simulink model "sm_boom_lift_crawler"  (R2026a)
settings: Solver=ode23t  StopTime=tVec.StopTime  FixedStep=2e-3  MaxStep=2  AbsTol=1e-3
StartFcn:
  | tic;
StopFcn:
  | Elapsed_Sim_Time = toc;
  | %disp(['Elapsed Sim Time = ' num2str(Elapsed_Sim_Time)]);
undefined symbols (not defined in the file): BasketR, Boom, Chassis, Extend, Jib, LevelM, LevelS, Lift, operator_seq, OutFL, OutFR, OutRL, OutRR, oVec, Tilt, TrackL, TrackR, Turret, tVec
libraries: sm_boom_lift_crawler_lib x14, nesl_utility x2, sm_lib x2, sm_boom_lift_crawler_lib_actuators x1, sm_boom_lift_crawler_lib_control x1, sm_boom_lift_crawler_lib_lift x1
(part 1 of 2)
Description:
  | Boom Lift Crawler with Hydraulic Actuation
  | 
  | Copyright 2020-2026 The MathWorks, Inc.
settings Model: Creator=smiller  LastModifiedBy=smiller
settings SolverCC: MaxConsecutiveMinStep=10
settings DataIOCC: SignalLoggingName=logsout_sm_boom_lift_crawler
settings SimscapeCC: SimscapeNominalValues="[{\"value\":\"1\",\"unit\":\"A\"},{\"value\":\"nomval_psi\",\"unit\":\"psi\"},{\"value\":\"1\",\"unit\":\"cm^2\"},{\"value\":\"nomval_cmv3_s\",\"unit\":\"cm^3/s\"},{\"value\":\"1\",\"unit\":\"kJ/kg\"},{\"value\":\"1\",\"unit\":\"kW\"},{\"value\":\"1\",\"unit\":\"l\"},{\"value\":\"nomval_N\",\"unit\":\"N\"},{\"value\":\"nomval_Nm\",\"unit\":\"N*m\"},{\"value\":\"1\",\"unit\":\"V\"}]"  SimscapeLogName=simlog_sm_boom_lift_crawler  SimscapeLogLimitData=off  SimscapeLogDataHistory=5000.0  SimscapeUseOperatingPoints=on  SimscapeOperatingPoint=op_hold15Sec_FULL
settings DiagnosticsConfigSet: SimMechanicsConflictingReferenceFrames=none  SimMechanicsRigidlyBoundBlock=none  SimMechanicsUnsatisfiedHighPriorityTargets=none
settings ExplorerConfigSet: InternalSimMechanicsExplorerSettings="<ExplorerConfiguration><canonicalview>default</canonicalview><AnimationSetting><BasePlaybackSpeed>1.0</BasePlaybackSpeed><PlaybackSpeedFactor>8.0</PlaybackSpeedFactor></AnimationSetting><TilePanel><TileInfo><Tiles Columns=\"1\" Count=\"1\" Rows=\"1\"><Column Weight=\"1\"/><Row Weight=\"1\"/><Tile Height=\"1\" Width=\"1\" X=\"0\" Y=\"0\"/></Tiles></TileInfo><SceneInfo><SceneViewer><BGColor><R>1</R><G>1</G><B>1</B></BGColor><Camera><DoPerspective>on</DoPerspective><Position><X>-12.2424581714389937</X><Y>-0.143345264209557399</Y><Z>4.1505972342390427</Z></Position><Center><X>-4.62122899968606404</X><Y>-0.143345264209557399</Y><Z>4.15059723423904359</Z></Center><Up><X>0</X><Y>0</Y><Z>1</Z></Up><ViewLimDist>1</ViewLimDist><YLim>0.466307658154998583</YLim><XLim>0.828991392275552963</XLim></Camera></SceneViewer></SceneInfo></TilePanel><MechEditorPanel><Cameras><Camera><Id>Camera8</Id><Value><Name>Extend_Knuckle</Name><NativeCamera><PositionTrackingFeature>Lift.Boom.Arms.Telescope.Extend_Cylinder.Transform_Camera_Extend_Knuckle.F</PositionTrackingFeature><CenterTrackingFeature>Lift.Boom.Arms.Telescope.Extend_Cylinder.Transform_Camera_Extend_Knuckle.F</CenterTrackingFeature><UpVectorTrackingFeature>Lift.Boom.Arms.Telescope.Extend_Cylinder.Transform_Camera_Extend_Knuckle.F</UpVectorTrackingFeature><CenterTrackingOrigin>off</CenterTrackingOrigin><CenterTrackingDirection>-X</CenterTrackingDirection><UpVectorTrackingDirection>-Y</UpVectorTrackingDirection></NativeCamera></Value></Camera><Camera><Id>Camera9</Id><Value><Name>Extend_Basket</Name><NativeCamera><PositionTrackingFeature>Lift.Boom.Arms.Telescope.Extend_Cylinder.Transform_Camera_Extend_Basket.F</PositionTrackingFeature><CenterTrackingFeature>Lift.Boom.Arms.Telescope.Extend_Cylinder.Transform_Camera_Extend_Basket.F</CenterTrackingFeature><UpVectorTrackingFeature>Lift.Boom.Arms.Telescope.Extend_Cylinder.Transform_Camera_Extend_Basket.F</UpVectorTrackingFeature><CenterTrackingOrigin>off</CenterTrackingOrigin><CenterTrackingDirection>+X</CenterTrackingDirection><UpVectorTrackingDirection>+Y</UpVectorTrackingDirection></NativeCamera></Value></Camera><Camera><Id>Camera10</Id><Value><Name>Basket_Rotate</Name><NativeCamera><PositionTrackingFeature>Lift.Boom.Basket.Basket_Rotate.Bracket.Reference_Camera_Basket_Rotate_L.R</PositionTrackingFeature><CenterTrackingFeature>Lift.Boom.Basket.Basket_Rotate.Bracket.Reference_Camera_Basket_Rotate_L.R</CenterTrackingFeature><UpVectorTrackingFeature>Mech_Config.World.W</UpVectorTrackingFeature><CenterTrackingOrigin>off</CenterTrackingOrigin><CenterTrackingDirection>-X</CenterTrackingDirection><UpVectorTrackingDirection>+Z</UpVectorTrackingDirection></NativeCamera></Value></Camera><Camera><Id>Camera11</Id><Value><Name>Tilt_Knuckle</Name><NativeCamera><PositionTrackingFeature>Lift.Boom.Arms.Tower.Upper_Knuckle.Reference_Knuckle_Cam.R</PositionTrackingFeature><CenterTrackingFeature>Lift.Boom.Arms.Tower.Upper_Knuckle.Reference_Knuckle_Cam.R</CenterTrackingFeature><UpVectorTrackingFeature>Mech_Config.World.W</UpVectorTrackingFeature><CenterTrackingOrigin>off</CenterTrackingOrigin><CenterTrackingDirection>+Z</CenterTrackingDirection><UpVectorTrackingDirection>+Z</UpVectorTrackingDirection></NativeCamera></Value></Camera><Camera><Id>Camera12</Id><Value><Name>Full Test</Name><NativeCamera><PositionKeyframeSet><Keyframe><Time>0</Time><Value><X>-12.242458171438994</X><Y>-0.1433452642095574</Y><Z>4.1505972342390427</Z></Value></Keyframe><Keyframe><Time>69.026826430124729</Time><Value><X>-14.974593328379619</X><Y>0.0056652615564253064</Y><Z>5.3389029552684786</Z></Value></Keyframe><Keyframe><Time>110.29539843687829</Time><Value><X>-21.00761369699504</X><Y>-0.0057417156870510078</Y><Z>8.0689402037867488</Z></Value></Keyframe><Keyframe><Time>140.70430157635164</Time><Value><X>-31.272784439198116</X><Y>-2.5583130214499052e-10</Y><Z>12.723321478963756</Z></Value></Keyframe><Keyframe><Time>181.77628976806102</Time><Value><X>-31.272784439198116</X><Y>-2.5583130214499052e-10</Y><Z>12.723321478963756</Z></Value></Keyframe><Keyframe><Time>208.0087867386398</Time><Value><X>-23.351505250921551</X><Y>-2.5583182919801497e-10</Y><Z>9.1371534281977738</Z></Value></Keyframe><Keyframe><Time>243.06358572448306</Time><Value><X>-16.577121762622586</X><Y>-2.5583144573665537e-10</Y><Z>6.0702143126734844</Z></Value></Keyframe><Keyframe><Time>273.3415757110605</Time><Value><X>-16.577121762622586</X><Y>-2.5583144573665537e-10</Y><Z>6.0702143126734844</Z></Value></Keyframe><Keyframe><Time>321.2447002217541</Time><Value><X>-13.690590902490033</X><Y>0.01787769923724114</Y><Z>4.7891626503614262</Z></Value></Keyframe><Keyframe><Time>350</Time><Value><X>-13.690590902490033</X><Y>0.01787769923724114</Y><Z>4.7891626503614262</Z></Value></Keyframe></PositionKeyframeSet><CenterKeyframeSet><Keyframe><Time>0</Time><Value><X>-4.621228999686064</X><Y>-0.1433452642095574</Y><Z>4.1505972342390436</Z></Value></Keyframe><Keyframe><Time>69.026826430124729</Time><Value><X>-0.17395018713353672</X><Y>0.0056652615564253064</Y><Z>5.3389029552684786</Z></Value></Keyframe><Keyframe><Time>110.29539843687829</Time><Value><X>-9.0038066291239502</X><Y>-0.0057417156870549491</Y><Z>8.0689402037867524</Z></Value></Keyframe><Keyframe><Time>140.70430157635164</Time><Value><X>-14.136391845814327</X><Y>-2.5583979379462107e-10</Y><Z>12.72332147896376</Z></Value></Keyframe><Keyframe><Time>181.77628976806102</Time><Value><X>-2.3429975002054775</X><Y>-2.5584563781180217e-10</Y><Z>12.723321478963761</Z></Value></Keyframe><Keyframe><Time>208.0087867386398</Time><Value><X>-10.17575261115104</X><Y>-2.5583801743778167e-10</Y><Z>9.1371534281977755</Z></Value></Keyframe><Keyframe><Time>243.06358572448306</Time><Value><X>-0.54476849060194255</X><Y>-2.5583897563257738e-10</Y><Z>6.0702143126734844</Z></Value></Keyframe><Keyframe><Time>273.3415757110605</Time><Value><X>-0.11057247639663359</X><Y>-2.5583917956089291e-10</Y><Z>6.0702143126734844</Z></Value></Keyframe><Keyframe><Time>321.2447002217541</Time><Value><X>-5.3452949964231387</X><Y>0.017877699237237366</Y><Z>4.7891626503614253</Z></Value></Keyframe><Keyframe><Time>350</Time><Value><X>-5.3452949964231387</X><Y>0.017877699237237366</Y><Z>4.7891626503614253</Z></Value></Keyframe></CenterKeyframeSet><UpVectorKeyframeSet><Keyframe><Time>0</Time><Value><X>0</X><Y>0</Y><Z>1</Z></Value></Keyframe><Keyframe><Time>69.026826430124729</Time><Value><X>0</X><Y>0</Y><Z>1</Z></Value></Keyframe><Keyframe><Time>110.29539843687829</Time><Value><X>0</X><Y>0</Y><Z>1</Z></Value></Keyframe><Keyframe><Time>140.70430157635164</Time><Value><X>0</X><Y>0</Y><Z>1</Z></Value></Keyframe><Keyframe><Time>181.77628976806102</Time><Value><X>-2.0731981129868445e-16</X><Y>1.0273382740432149e-31</Y><Z>1</Z></Value></Keyframe><Keyframe><Time>208.0087867386398</Time><Value><X>1.4663775813922931e-57</X><Y>2.9591920320379324e-42</Y><Z>1</Z></Value></Keyframe><Keyframe><Time>243.06358572448306</Time><Value><X>1.3898401336634517e-57</X><Y>2.9591920320379324e-42</Y><Z>1</Z></Value></Keyframe><Keyframe><Time>273.3415757110605</Time><Value><X>1.3898401336605064e-57</X><Y>2.9591920320379324e-42</Y><Z>1</Z></Value></Keyframe><Keyframe><Time>321.2447002217541</Time><Value><X>1.3198478700492623e-57</X><Y>2.9591920320379324e-42</Y><Z>1</Z></Value></Keyframe><Keyframe><Time>350</Time><Value><X>1.0642863113510858e-16</X><Y>-4.813997747953607e-32</Y><Z>1</Z></Value></Keyframe></UpVectorKeyframeSet></NativeCamera></Value></Camera><Camera><Id>Camera13</Id><Value><Name>View_Basket_World</Name><NativeCamera><PositionTrackingFeature>Lift.Boom.Basket.Basket.Reference_Basket_Cam.R</PositionTrackingFeature><CenterTrackingFeature>Mech_Config.World.W</CenterTrackingFeature><UpVectorTrackingFeature>Lift.Boom.Basket.Basket.Reference_Basket_Cam.R</UpVectorTrackingFeature><CenterTrackingOrigin>on</CenterTrackingOrigin><UpVectorTrackingDirection>+Y</UpVectorTrackingDirection></NativeCamera></Value></Camera><Camera><Id>Camera14</Id><Value><Name>View_Worm_Drive</Name><NativeCamera><PositionTrackingFeature>Lift.Boom.Turret.Case.Reference_Worm_Cam.R</PositionTrackingFeature><CenterTrackingFeature>Lift.Boom.Turret.Case.Transform_Worm_Cam.B</CenterTrackingFeature><UpVectorTrackingFeature>Mech_Config.World.W</UpVectorTrackingFeature><CenterTrackingOrigin>on</CenterTrackingOrigin><UpVectorTrackingDirection>+Z</UpVectorTrackingDirection></NativeCamera></Value></Camera><Camera><Id>Camera15</Id><Value><Name>Extend_Retract_Pulley</Name><NativeCamera><PositionTrackingFeature>Lift.Boom.Arms.Telescope.Extend_Cylinder.Reference_Camera_Retract_Pulley.R</PositionTrackingFeature><CenterTrackingFeature>Lift.Boom.Arms.Telescope.Extend_Cylinder.Reference_Camera_Retract_Pulley.R</CenterTrackingFeature><UpVectorTrackingFeature>Lift.Boom.Arms.Telescope.Extend_Cylinder.Reference_Camera_Retract_Pulley.R</UpVectorTrackingFeature><CenterTrackingOrigin>off</CenterTrackingOrigin><CenterTrackingDirection>+Y</CenterTrackingDirection><UpVectorTrackingDirection>+Z</UpVectorTrackingDirection></NativeCamera></Value></Camera><Camera><Id>Camera16</Id><Value><Name>Extend_Extend_Pulley</Name><NativeCamera><PositionTrackingFeature>Lift.Boom.Arms.Telescope.Extend_Cylinder.Reference_Camera_Extend_Pulley.R</PositionTrackingFeature><CenterTrackingFeature>Lift.Boom.Arms.Telescope.Extend_Cylinder.Reference_Camera_Extend_Pulley.R</CenterTrackingFeature><UpVectorTrackingFeature>Lift.Boom.Arms.Telescope.Extend_Cylinder.Reference_Camera_Extend_Pulley.R</UpVectorTrackingFeature><CenterTrackingOrigin>off</CenterTrackingOrigin><CenterTrackingDirection>+Z</CenterTrackingDirection><UpVectorTrackingDirection>-Y</UpVectorTrackingDirection></NativeCamera></Value></Camera><Camera><Id>Camera17</Id><Value><Name>Jib</Name><NativeCamera><PositionTrackingFeature>Lift.Boom.Basket.Jib.Jib_Mount.Reference_Camera_Basket_Jib.R</PositionTrackingFeature><CenterTrackingFeature>Lift.Boom.Basket.Jib.Jib_Mount.Reference_Camera_Basket_Jib.R</CenterTrackingFeature><UpVectorTrackingFeature>Mech_Config.World.W</UpVectorTrackingFeature><CenterTrackingOrigin>off</CenterTrackingOrigin><CenterTrackingDirection>-X</CenterTrackingDirection><UpVectorTrackingDirection>+Z</UpVectorTrackingDirection></NativeCamera></Value></Camera></Cameras><GfxPanelCameraMap><MapElement CameraMLId=\"Camera12\" GfxPanelIndex=\"0\"/></GfxPanelCameraMap><VideoCreator><PlaybackSpeedRatio>8</PlaybackSpeedRatio><FrameRate>30</FrameRate><VideoFormat>MPEG-4</VideoFormat><FrameSize>auto</FrameSize></VideoCreator></MechEditorPanel></ExplorerConfiguration>"

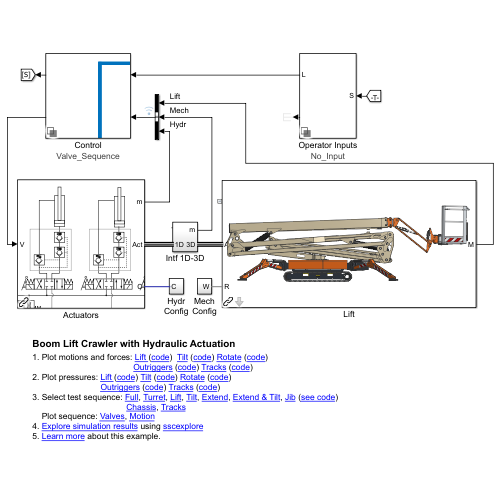
[thumbnail: Simulink's stored preview of the top-level diagram]
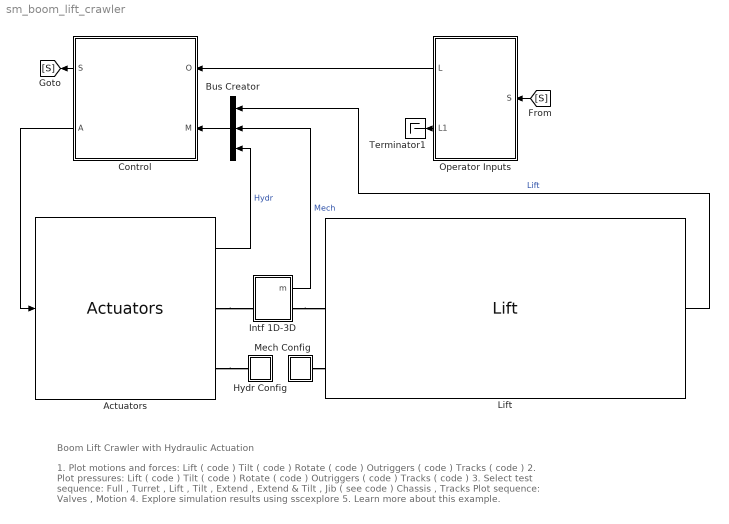
== system sm_boom_lift_crawler ==
  note: 1. Plot motions and forces: Lift ( code ) Tilt ( code ) Rotate ( code )
      | Outriggers ( code ) Tracks ( code )
      | 2. Plot pressures: Lift ( code ) Tilt ( code ) Rotate ( code )
      | Outriggers ( code ) Tracks ( code )
      | 3. Select test sequence: Full , Turret , Lift , Tilt , Extend , Extend & Tilt , Jib ( see code )
      | Chassis , Tracks
      | Plot sequence: Valves , Motion
      | 4. Explore simulation results using sscexplore
      | 5. Learn more about this example.
  note: Boom Lift Crawler with Hydraulic Actuation
  Actuators : sm_boom_lift_crawler_lib_actuators/Actuators  SystemSampleTime=-1  VariantControl=Actuators_CVs  VariantActivationTime=update diagram  EmptyChoice=off  PassThrough=off  PassThroughVariantControl=(default)  EmptyChoiceVariantControl=(default)  AllowFlexibleInterface=on  Latency=0  AutoFrameSizeCalculation=off
  Bus Creator : BusCreator  Inputs=3
  Control : Subsystem  Variant=on  VariantControlMode=label  VariantControl=Variant1  LabelModeActiveChoice=Valve_Sequence
      settings: AttributesFormatString=%<LabelModeActiveChoice>
      mask Display:
      | blk = sm_boom_lift_activeVariantBlock(gcb);
      | eval(get_param(blk, 'MaskDisplay'));
  Hydr Config : Subsystem
  Intf 1D-3D : Subsystem
  Lift : sm_boom_lift_crawler_lib_lift/Lift  popup_gnd_outr=Force
  Mech Config : Subsystem
  Operator Inputs : Subsystem  Variant=on  VariantControlMode=label  VariantControl=Variant1  LabelModeActiveChoice=No_Input
      settings: AttributesFormatString=%<LabelModeActiveChoice>
      mask Display:
      | blk = sm_boom_lift_activeVariantBlock(gcb);
      | eval(get_param(blk, 'MaskDisplay'));
  Terminator1 : Terminator
  wires:
  Control/2(A) -> Actuators/1
  Operator Inputs/1(L) -> Control/1(O)
  Actuators/1 -> Bus Creator/3  "Hydr"
  Intf 1D-3D/1(m) -> Bus Creator/2  "Mech"
  Bus Creator/1 -> Control/2(M)
  Lift/1 -> Bus Creator/1  "Lift"
  Operator Inputs/2(L1) -> Terminator1/1
  [S] -> Operator Inputs/1(S)
  Control/1(S) -> [S]
  connections:
  Mech Config/LConn1 -- Lift/LConn3
  Intf 1D-3D/RConn1 -- Lift/LConn2
  Actuators/RConn1 -- Intf 1D-3D/LConn2
  Actuators/RConn2 -- Hydr Config/RConn1

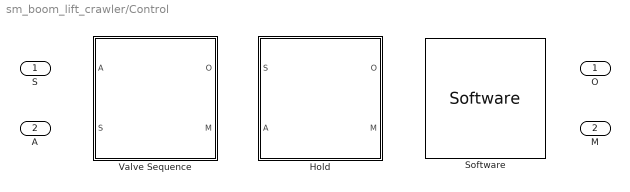
== system sm_boom_lift_crawler/Control ==
  O : Inport
  M : Inport  Port=2
  Hold : Subsystem  VariantControl=Hold
      mask Display: image('sm_boom_lift_crawler_valve_seq_hold.svg');
  Software : sm_boom_lift_crawler_lib_control/Software  SystemSampleTime=-1  VariantControl=Software  VariantActivationTime=update diagram  EmptyChoice=off  PassThrough=off  PassThroughVariantControl=(default)  EmptyChoiceVariantControl=(default)  AllowFlexibleInterface=on  Latency=0  AutoFrameSizeCalculation=off
  Valve Sequence : Subsystem  VariantControl=Valve_Sequence
      mask Display: image('sm_boom_lift_crawler_valve_seq.svg');
  S : Outport
  A : Outport  Port=2

== system sm_boom_lift_crawler/Hydr Config ==
  Solver Configuration : nesl_utility/Solver Configuration  PhysicalDomain=network_engine_domain  SubClassName=solver  LeftPortType=input  RightPortType=generic  Tones=[]  Harmonics=[]  SimulateNoise=off  Profile=off  UseLocalSampling=off  EnableSwitchedLinearOptims=on  FrequencyDomain=off  UseCCode=off  RelTol=0.001  AbsTol=1e-06  MinStep=1e-09  ToWorkspace=off  RevertToSquareIcSolve=off  NumHomotopyIterations=100  PhasorMode=off  PhasorModeNumHarmonics=1  ConsistencySolver=NEWTON_FTOL  CanonicalOrdering=UNORDERED  OptimizeIntermediates=UNOPTIMIZED  IndexReductionMethod=DerivativeReplacement  DoDC=off  ResidualTolerance=1e-9  ConsistencyTolSource=GLOBAL  ConsistencyAbsTol=0.001  ConsistencyRelTol=0.001  ConsistencyTolFactor=0.001  UseLocalSolver=off  LocalSolverChoice=NE_PARTITIONING_ADVANCER  ResolveIndetEquations=on  FunctionEvalNumThread=1  LocalSolverSampleTime=1e-3 %2e-3  DoFixedCost=off  MaxNonlinIter=10  MaxModeIter=2  ComputeImpulses=off  ImpulseIterations=2  LinearAlgebra=Sparse  LinearAlgebraNumThread=0  EquationFormulation=NE_TIME_EF  DelaysMemoryBudget=1024  AutomaticFiltering=on  FilteringTimeConstant=1e-3  PartitionStorageMethod=EXHAUSTIVE  PartitionMemoryBudget=1024  PartitionMethod=ROBUST  MultibodyUseLocalSolver=off  MultibodyLocalSolverChoice=ODE1  MultibodyLocalSolverSampleTime=0.001
  C : PMIOPort  Side=Right
  connections:
  C/RConn1 -- Solver Configuration/RConn1

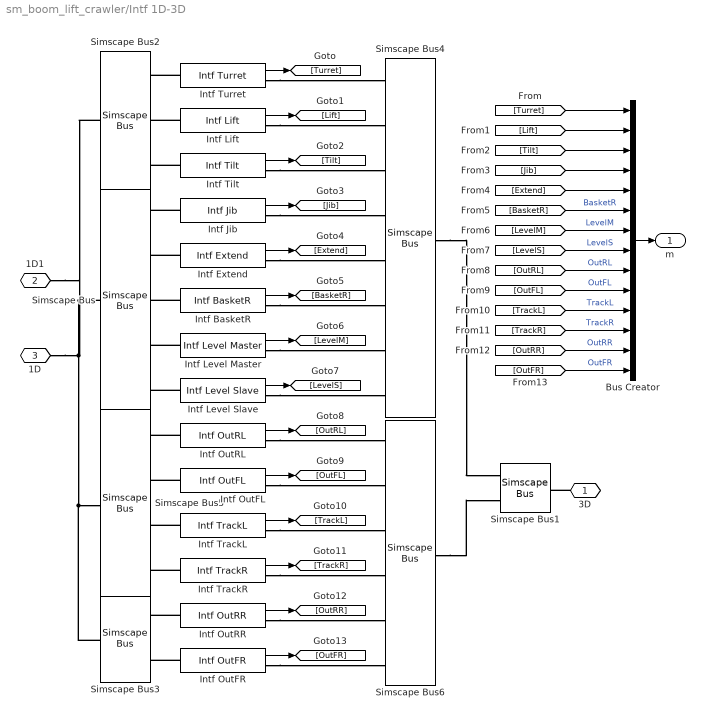
== system sm_boom_lift_crawler/Intf 1D-3D ==
  Bus Creator : BusCreator  Inputs=14
  Intf BasketR : sm_boom_lift_crawler_lib/Intf BasketR  SystemSampleTime=-1  VariantActivationTime=update diagram  EmptyChoice=off  PassThrough=off  PassThroughVariantControl=(default)  EmptyChoiceVariantControl=(default)  AllowFlexibleInterface=on  Latency=0  AutoFrameSizeCalculation=off
  Intf Extend : sm_boom_lift_crawler_lib/Intf Extend  SystemSampleTime=-1  VariantActivationTime=update diagram  EmptyChoice=off  PassThrough=off  PassThroughVariantControl=(default)  EmptyChoiceVariantControl=(default)  AllowFlexibleInterface=on  Latency=0  AutoFrameSizeCalculation=off
  Intf Jib : sm_boom_lift_crawler_lib/Intf Jib  SystemSampleTime=-1  VariantActivationTime=update diagram  EmptyChoice=off  PassThrough=off  PassThroughVariantControl=(default)  EmptyChoiceVariantControl=(default)  AllowFlexibleInterface=on  Latency=0  AutoFrameSizeCalculation=off
  Intf Level Master : sm_boom_lift_crawler_lib/Intf Level Master  SystemSampleTime=-1  VariantActivationTime=update diagram  EmptyChoice=off  PassThrough=off  PassThroughVariantControl=(default)  EmptyChoiceVariantControl=(default)  AllowFlexibleInterface=on  Latency=0  AutoFrameSizeCalculation=off
  Intf Level Slave : sm_boom_lift_crawler_lib/Intf Level Slave  SystemSampleTime=-1  VariantActivationTime=update diagram  EmptyChoice=off  PassThrough=off  PassThroughVariantControl=(default)  EmptyChoiceVariantControl=(default)  AllowFlexibleInterface=on  Latency=0  AutoFrameSizeCalculation=off
  Intf Lift : sm_boom_lift_crawler_lib/Intf Lift  SystemSampleTime=-1  VariantActivationTime=update diagram  EmptyChoice=off  PassThrough=off  PassThroughVariantControl=(default)  EmptyChoiceVariantControl=(default)  AllowFlexibleInterface=on  Latency=0  AutoFrameSizeCalculation=off
  Intf OutFL : sm_boom_lift_crawler_lib/Intf OutFL  SystemSampleTime=-1  VariantActivationTime=update diagram  EmptyChoice=off  PassThrough=off  PassThroughVariantControl=(default)  EmptyChoiceVariantControl=(default)  AllowFlexibleInterface=on  Latency=0  AutoFrameSizeCalculation=off
  Intf OutFR : sm_boom_lift_crawler_lib/Intf OutFR  SystemSampleTime=-1  VariantActivationTime=update diagram  EmptyChoice=off  PassThrough=off  PassThroughVariantControl=(default)  EmptyChoiceVariantControl=(default)  AllowFlexibleInterface=on  Latency=0  AutoFrameSizeCalculation=off
  Intf OutRL : sm_boom_lift_crawler_lib/Intf OutRL  SystemSampleTime=-1  VariantActivationTime=update diagram  EmptyChoice=off  PassThrough=off  PassThroughVariantControl=(default)  EmptyChoiceVariantControl=(default)  AllowFlexibleInterface=on  Latency=0  AutoFrameSizeCalculation=off
  Intf OutRR : sm_boom_lift_crawler_lib/Intf OutRR  SystemSampleTime=-1  VariantActivationTime=update diagram  EmptyChoice=off  PassThrough=off  PassThroughVariantControl=(default)  EmptyChoiceVariantControl=(default)  AllowFlexibleInterface=on  Latency=0  AutoFrameSizeCalculation=off
  Intf Tilt : sm_boom_lift_crawler_lib/Intf Tilt  SystemSampleTime=-1  VariantActivationTime=update diagram  EmptyChoice=off  PassThrough=off  PassThroughVariantControl=(default)  EmptyChoiceVariantControl=(default)  AllowFlexibleInterface=on  Latency=0  AutoFrameSizeCalculation=off
  Intf TrackL : sm_boom_lift_crawler_lib/Intf TrackL  SystemSampleTime=-1  VariantActivationTime=update diagram  EmptyChoice=off  PassThrough=off  PassThroughVariantControl=(default)  EmptyChoiceVariantControl=(default)  AllowFlexibleInterface=on  Latency=0  AutoFrameSizeCalculation=off
  Intf TrackR : sm_boom_lift_crawler_lib/Intf TrackR  SystemSampleTime=-1  VariantActivationTime=update diagram  EmptyChoice=off  PassThrough=off  PassThroughVariantControl=(default)  EmptyChoiceVariantControl=(default)  AllowFlexibleInterface=on  Latency=0  AutoFrameSizeCalculation=off
  Intf Turret : sm_boom_lift_crawler_lib/Intf Turret  SystemSampleTime=-1  VariantActivationTime=update diagram  EmptyChoice=off  PassThrough=off  PassThroughVariantControl=(default)  EmptyChoiceVariantControl=(default)  AllowFlexibleInterface=on  Latency=0  AutoFrameSizeCalculation=off
  Simscape Bus : SimscapeBus  HierarchyStrings=Jib;Extend;BasketR;LevelM;LevelS
  Simscape Bus1 : SimscapeBus  HierarchyStrings=Boom;Chassis
  Simscape Bus2 : SimscapeBus  HierarchyStrings=Turret;Lift;Tilt
  Simscape Bus3 : SimscapeBus  HierarchyStrings=OutRR;OutFR
  Simscape Bus4 : SimscapeBus  HierarchyStrings=Turret;Lift;Tilt;Jib;Extend;BasketR;LevelM;LevelS
  Simscape Bus5 : SimscapeBus  HierarchyStrings=OutRL;OutFL;TrackL;TrackR
  Simscape Bus6 : SimscapeBus  HierarchyStrings=OutRL;OutFL;TrackL;TrackR;OutRR;OutFR
  3D : PMIOPort  Side=Right
  1D1 : PMIOPort  Port=2  Side=Left
  1D : PMIOPort  Port=3  Side=Left
  m : Outport
  wires:
  Intf OutFR/1 -> [OutFR]
  Intf OutRR/1 -> [OutRR]
  Intf TrackR/1 -> [TrackR]
  Intf TrackL/1 -> [TrackL]
  Intf OutFL/1 -> [OutFL]
  Intf OutRL/1 -> [OutRL]
  Intf Level Slave/1 -> [LevelS]
  Intf Level Master/1 -> [LevelM]
  Intf BasketR/1 -> [BasketR]
  Intf Extend/1 -> [Extend]
  Intf Jib/1 -> [Jib]
  Intf Tilt/1 -> [Tilt]
  Intf Lift/1 -> [Lift]
  Intf Turret/1 -> [Turret]
  [OutFR] -> Bus Creator/14  "OutFR"
  [OutRR] -> Bus Creator/13  "OutRR"
  [Extend] -> Bus Creator/5
  [OutRL] -> Bus Creator/9  "OutRL"
  [TrackL] -> Bus Creator/11  "TrackL"
  [LevelM] -> Bus Creator/7  "LevelM"
  [Turret] -> Bus Creator/1
  [OutFL] -> Bus Creator/10  "OutFL"
  [Tilt] -> Bus Creator/3
  [Lift] -> Bus Creator/2
  [TrackR] -> Bus Creator/12  "TrackR"
  [LevelS] -> Bus Creator/8  "LevelS"
  Bus Creator/1 -> m/1
  [Jib] -> Bus Creator/4
  [BasketR] -> Bus Creator/6  "BasketR"
  connections:
  Intf OutRR/RConn1 -- Simscape Bus6/LConn5
  Intf OutRR/LConn1 -- Simscape Bus3/LConn1
  Intf OutFR/RConn1 -- Simscape Bus6/LConn6
  Intf OutFR/LConn1 -- Simscape Bus3/LConn2
  Intf TrackR/RConn1 -- Simscape Bus6/LConn4
  Intf TrackR/LConn1 -- Simscape Bus5/LConn4
  Intf TrackL/RConn1 -- Simscape Bus6/LConn3
  Intf TrackL/LConn1 -- Simscape Bus5/LConn3
  Intf OutRL/LConn1 -- Simscape Bus5/LConn1
  Intf OutRL/RConn1 -- Simscape Bus6/LConn1
  Intf OutFL/LConn1 -- Simscape Bus5/LConn2
  Intf OutFL/RConn1 -- Simscape Bus6/LConn2
  Simscape Bus6/RConn1 -- Simscape Bus1/LConn2
  Simscape Bus3/RConn1 -- Simscape Bus5/RConn1 -- 1D/RConn1 -- Simscape Bus2/RConn1 -- 1D1/RConn1 -- Simscape Bus/RConn1
  Intf Level Slave/RConn1 -- Simscape Bus4/LConn8
  Intf Level Slave/LConn1 -- Simscape Bus/LConn5
  Intf Level Master/RConn1 -- Simscape Bus4/LConn7
  Intf Level Master/LConn1 -- Simscape Bus/LConn4
  Intf BasketR/RConn1 -- Simscape Bus4/LConn6
  Intf BasketR/LConn1 -- Simscape Bus/LConn3
  Intf Extend/RConn1 -- Simscape Bus4/LConn5
  Intf Extend/LConn1 -- Simscape Bus/LConn2
  Intf Jib/LConn1 -- Simscape Bus/LConn1
  Intf Jib/RConn1 -- Simscape Bus4/LConn4
  Intf Tilt/RConn1 -- Simscape Bus4/LConn3
  Intf Tilt/LConn1 -- Simscape Bus2/LConn3
  Intf Lift/LConn1 -- Simscape Bus2/LConn2
  Intf Lift/RConn1 -- Simscape Bus4/LConn2
  Intf Turret/RConn1 -- Simscape Bus4/LConn1
  Intf Turret/LConn1 -- Simscape Bus2/LConn1
  Simscape Bus4/RConn1 -- Simscape Bus1/LConn1
  3D/RConn1 -- Simscape Bus1/RConn1

== system sm_boom_lift_crawler/Mech Config ==
  Mechanism Configuration : sm_lib/Utilities/Mechanism Configuration  UniformGravity=Constant  GravityVector=[0 0 -9.80665]  GravityVectorUnits=m/s^2  LinearizationDelta=0.001  JointModeTransitionNonlinearIterations=2
  Solver Configuration : nesl_utility/Solver Configuration  PhysicalDomain=network_engine_domain  SubClassName=solver  LeftPortType=input  RightPortType=generic  Tones=[]  Harmonics=[]  SimulateNoise=off  Profile=off  UseLocalSampling=off  EnableSwitchedLinearOptims=on  FrequencyDomain=off  UseCCode=off  RelTol=0.001  AbsTol=1e-06  MinStep=1e-09  ToWorkspace=off  RevertToSquareIcSolve=off  NumHomotopyIterations=100  PhasorMode=off  PhasorModeNumHarmonics=1  ConsistencySolver=NEWTON_FTOL  CanonicalOrdering=UNORDERED  OptimizeIntermediates=UNOPTIMIZED  IndexReductionMethod=DerivativeReplacement  DoDC=off  ResidualTolerance=1e-9  ConsistencyTolSource=GLOBAL  ConsistencyAbsTol=0.001  ConsistencyRelTol=0.001  ConsistencyTolFactor=0.001  UseLocalSolver=off  LocalSolverChoice=NE_BACKWARD_EULER_ADVANCER  ResolveIndetEquations=on  FunctionEvalNumThread=1  LocalSolverSampleTime=2e-3  DoFixedCost=off  MaxNonlinIter=3  MaxModeIter=2  ComputeImpulses=off  ImpulseIterations=2  LinearAlgebra=auto  LinearAlgebraNumThread=0  EquationFormulation=NE_TIME_EF  DelaysMemoryBudget=1024  AutomaticFiltering=on  FilteringTimeConstant=0.001  PartitionStorageMethod=AS_NEEDED  PartitionMemoryBudget=1024  PartitionMethod=ROBUST  MultibodyUseLocalSolver=off  MultibodyLocalSolverChoice=ODE1  MultibodyLocalSolverSampleTime=0.001
  World : sm_lib/Frames and Transforms/World Frame
  W : PMIOPort  Side=Left
  connections:
  Solver Configuration/RConn1 -- W/RConn1 -- Mechanism Configuration/RConn1 -- World/RConn1

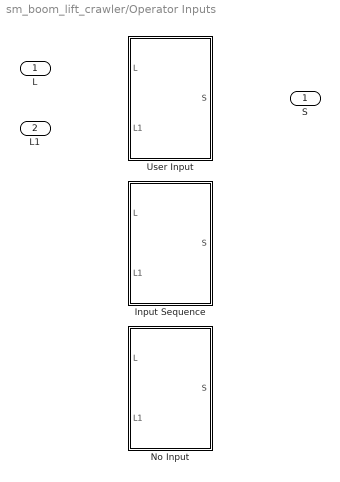
== system sm_boom_lift_crawler/Operator Inputs ==
  S : Inport
  Input Sequence : Subsystem  VariantControl=Input_Sequence
      mask Display: image('sm_boom_lift_crawler_operator_seq.svg');
  No Input : Subsystem  VariantControl=No_Input
      mask Display: %image('sl001_2x3.svg');
  User Input : Subsystem  VariantControl=User_Input
      mask Display: image('sl001_2x3.svg');
  L : Outport
  L1 : Outport  Port=2

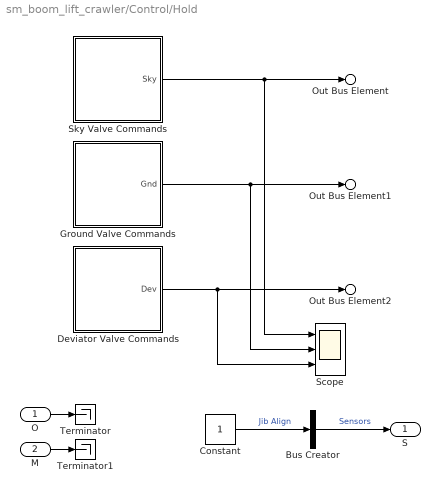
== system sm_boom_lift_crawler/Control/Hold ==
  O : Inport
  M : Inport  Port=2
  Bus Creator : BusCreator  Inputs=1
  Constant : Constant
  Deviator Valve Commands : Subsystem
  Ground Valve Commands : Subsystem
  Scope : Scope  NumInputPorts=3
      settings: ActiveDisplayYMinimum=-1  ActiveDisplayYMaximum=1
  Sky Valve Commands : Subsystem
  Terminator : Terminator
  Terminator1 : Terminator
  S : Outport
  Out Bus Element : Outport  Port=2  PortName=A  Element=Sky
  Out Bus Element1 : Outport  Port=2  PortName=A  Element=Gnd
  Out Bus Element2 : Outport  Port=2  PortName=A  Element=Dev
  wires:
  Deviator Valve Commands/1(Dev) -> Scope/3, Out Bus Element2/1
  Ground Valve Commands/1(Gnd) -> Scope/2, Out Bus Element1/1
  Sky Valve Commands/1(Sky) -> Out Bus Element/1, Scope/1
  M/1 -> Terminator1/1
  O/1 -> Terminator/1
  Bus Creator/1 -> S/1  "Sensors"
  Constant/1 -> Bus Creator/1  "Jib Align"

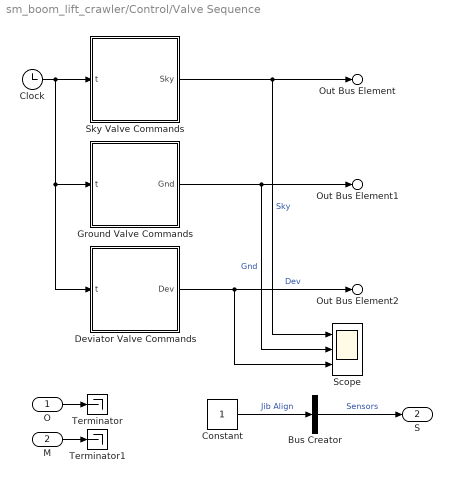
== system sm_boom_lift_crawler/Control/Valve Sequence ==
  O : Inport
  M : Inport  Port=2
  Bus Creator : BusCreator  Inputs=1
  Clock : Clock
  Constant : Constant
  Deviator Valve Commands : Subsystem
  Ground Valve Commands : Subsystem
  Scope : Scope  NumInputPorts=3
      settings: ActiveDisplayYMinimum=-1  ActiveDisplayYMaximum=1
  Sky Valve Commands : Subsystem
  Terminator : Terminator
  Terminator1 : Terminator
  Out Bus Element : Outport  PortName=A  Element=Sky
  Out Bus Element1 : Outport  PortName=A  Element=Gnd
  Out Bus Element2 : Outport  PortName=A  Element=Dev
  S : Outport  Port=2
  wires:
  Sky Valve Commands/1(Sky) -> Out Bus Element/1, Scope/1  "Sky"
  Ground Valve Commands/1(Gnd) -> Scope/2, Out Bus Element1/1  "Gnd"
  Clock/1 -> Deviator Valve Commands/1(t), Ground Valve Commands/1(t), Sky Valve Commands/1(t)
  Deviator Valve Commands/1(Dev) -> Out Bus Element2/1, Scope/3  "Dev"
  O/1 -> Terminator/1
  M/1 -> Terminator1/1
  Bus Creator/1 -> S/1  "Sensors"
  Constant/1 -> Bus Creator/1  "Jib Align"

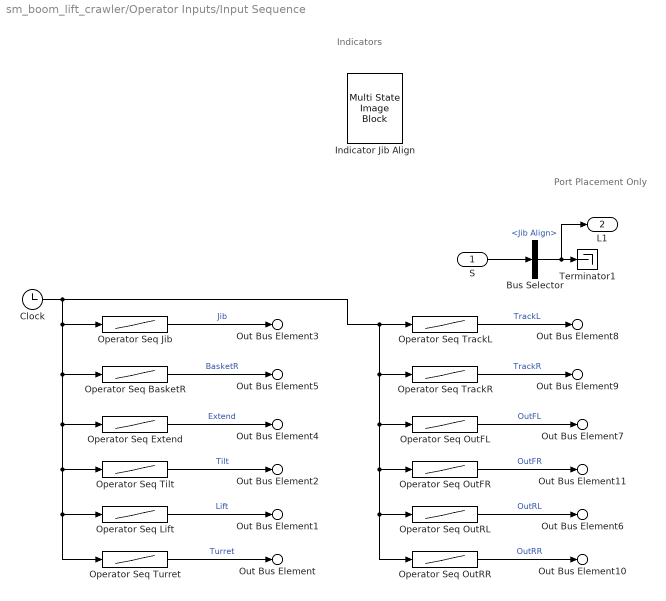
== system sm_boom_lift_crawler/Operator Inputs/Input Sequence ==
  note: Indicators
  note: Port
      | Placement
      | Only
  S : Inport
  Bus Selector : BusSelector  OutputSignals=Jib Align
  Clock : Clock
  Indicator Jib Align : MultiStateImageBlock
  Operator Seq BasketR : Lookup_n-D  NumberOfTableDimensions=1  BreakpointsForDimension1=operator_seq.basketR.t  Table=operator_seq.basketR.q  InterpMethod=Flat  ExtrapMethod=Clip  UseLastTableValue=on  InternalRulePriority=Speed  RndMeth=Simplest
  Operator Seq Extend : Lookup_n-D  NumberOfTableDimensions=1  BreakpointsForDimension1=operator_seq.extend.t  Table=operator_seq.extend.p  InterpMethod=Flat  ExtrapMethod=Clip  UseLastTableValue=on  InternalRulePriority=Speed  RndMeth=Simplest
  Operator Seq Jib : Lookup_n-D  NumberOfTableDimensions=1  BreakpointsForDimension1=operator_seq.jib.t  Table=operator_seq.jib.p  InterpMethod=Flat  ExtrapMethod=Clip  UseLastTableValue=on  InternalRulePriority=Speed  RndMeth=Simplest
  Operator Seq Lift : Lookup_n-D  NumberOfTableDimensions=1  BreakpointsForDimension1=operator_seq.lift.t  Table=operator_seq.lift.p  InterpMethod=Flat  ExtrapMethod=Clip  UseLastTableValue=on  InternalRulePriority=Speed  RndMeth=Simplest
  Operator Seq OutFL : Lookup_n-D  NumberOfTableDimensions=1  BreakpointsForDimension1=operator_seq.outFL.t  Table=operator_seq.outFL.p  InterpMethod=Flat  ExtrapMethod=Clip  UseLastTableValue=on  InternalRulePriority=Speed  RndMeth=Simplest
  Operator Seq OutFR : Lookup_n-D  NumberOfTableDimensions=1  BreakpointsForDimension1=operator_seq.outFR.t  Table=operator_seq.outFR.p  InterpMethod=Flat  ExtrapMethod=Clip  UseLastTableValue=on  InternalRulePriority=Speed  RndMeth=Simplest
  Operator Seq OutRL : Lookup_n-D  NumberOfTableDimensions=1  BreakpointsForDimension1=operator_seq.outRL.t  Table=operator_seq.outRL.p  InterpMethod=Flat  ExtrapMethod=Clip  UseLastTableValue=on  InternalRulePriority=Speed  RndMeth=Simplest
  Operator Seq OutRR : Lookup_n-D  NumberOfTableDimensions=1  BreakpointsForDimension1=operator_seq.outRR.t  Table=operator_seq.outRR.p  InterpMethod=Flat  ExtrapMethod=Clip  UseLastTableValue=on  InternalRulePriority=Speed  RndMeth=Simplest
  Operator Seq Tilt : Lookup_n-D  NumberOfTableDimensions=1  BreakpointsForDimension1=operator_seq.tilt.t  Table=operator_seq.tilt.p  InterpMethod=Flat  ExtrapMethod=Clip  UseLastTableValue=on  InternalRulePriority=Speed  RndMeth=Simplest
  Operator Seq TrackL : Lookup_n-D  NumberOfTableDimensions=1  BreakpointsForDimension1=operator_seq.TrackL.t  Table=operator_seq.TrackL.p  InterpMethod=Flat  ExtrapMethod=Clip  UseLastTableValue=on  InternalRulePriority=Speed  RndMeth=Simplest
  Operator Seq TrackR : Lookup_n-D  NumberOfTableDimensions=1  BreakpointsForDimension1=operator_seq.TrackR.t  Table=operator_seq.TrackR.p  InterpMethod=Flat  ExtrapMethod=Clip  UseLastTableValue=on  InternalRulePriority=Speed  RndMeth=Simplest
  Operator Seq Turret : Lookup_n-D  NumberOfTableDimensions=1  BreakpointsForDimension1=operator_seq.turret.t  Table=operator_seq.turret.q  InterpMethod=Flat  ExtrapMethod=Clip  UseLastTableValue=on  InternalRulePriority=Speed  RndMeth=Simplest
  Terminator1 : Terminator
  Out Bus Element : Outport  PortName=L  Element=Turret
  Out Bus Element1 : Outport  PortName=L  Element=Lift
  Out Bus Element2 : Outport  PortName=L  Element=Tilt
  Out Bus Element3 : Outport  PortName=L  Element=Jib
  Out Bus Element4 : Outport  PortName=L  Element=Extend
  Out Bus Element5 : Outport  PortName=L  Element=BasketR
  Out Bus Element6 : Outport  PortName=L  Element=OutRL
  Out Bus Element7 : Outport  PortName=L  Element=OutFL
  Out Bus Element8 : Outport  PortName=L  Element=TrackL
  Out Bus Element9 : Outport  PortName=L  Element=TrackR
  Out Bus Element10 : Outport  PortName=L  Element=OutRR
  Out Bus Element11 : Outport  PortName=L  Element=OutFR
  L1 : Outport  Port=2
  wires:
  Operator Seq TrackR/1 -> Out Bus Element9/1  "TrackR"
  Bus Selector/1 -> Terminator1/1, L1/1  "<Jib Align>"
  S/1 -> Bus Selector/1
  Operator Seq Extend/1 -> Out Bus Element4/1  "Extend"
  Operator Seq Turret/1 -> Out Bus Element/1  "Turret"
  Operator Seq Lift/1 -> Out Bus Element1/1  "Lift"
  Operator Seq Tilt/1 -> Out Bus Element2/1  "Tilt"
  Operator Seq OutFL/1 -> Out Bus Element7/1  "OutFL"
  Operator Seq BasketR/1 -> Out Bus Element5/1  "BasketR"
  Operator Seq Jib/1 -> Out Bus Element3/1  "Jib"
  Operator Seq OutRL/1 -> Out Bus Element6/1  "OutRL"
  Operator Seq OutFR/1 -> Out Bus Element11/1  "OutFR"
  Operator Seq OutRR/1 -> Out Bus Element10/1  "OutRR"
  Operator Seq TrackL/1 -> Out Bus Element8/1  "TrackL"
  Clock/1 -> Operator Seq TrackR/1, Operator Seq OutFL/1, Operator Seq OutFR/1, Operator Seq OutRL/1, Operator Seq OutRR/1, Operator Seq TrackL/1, Operator Seq Jib/1, Operator Seq BasketR/1, Operator Seq Extend/1, Operator Seq Tilt/1, Operator Seq Lift/1, Operator Seq Turret/1

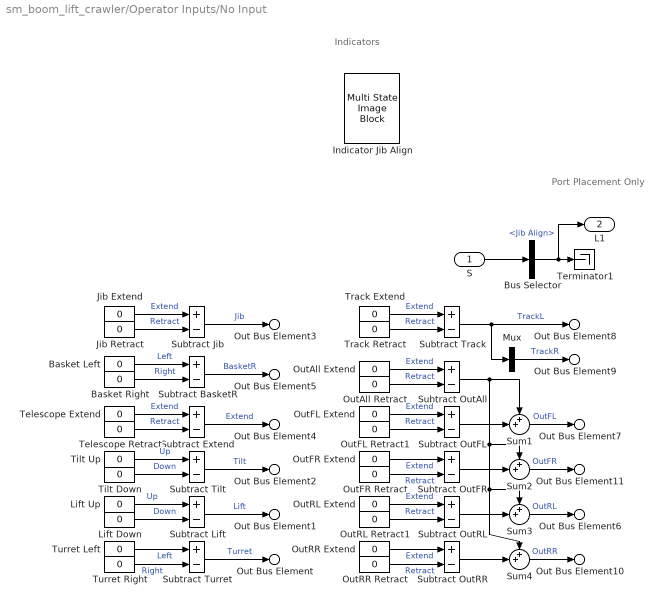
== system sm_boom_lift_crawler/Operator Inputs/No Input ==
  note: Indicators
  note: Port
      | Placement
      | Only
  S : Inport
  Basket Left : Constant  Value=0
  Basket Right : Constant  Value=0
  Bus Selector : BusSelector  OutputSignals=Jib Align
  Indicator Jib Align : MultiStateImageBlock
  Jib Extend : Constant  Value=0
  Jib Retract : Constant  Value=0
  Lift Down : Constant  Value=0
  Lift Up : Constant  Value=0
  Mux : Mux  Inputs=1
  OutAll Extend : Constant  Value=0
  OutAll Retract : Constant  Value=0
  OutFL Extend : Constant  Value=0
  OutFL Retract1 : Constant  Value=0
  OutFR Extend : Constant  Value=0
  OutFR Retract : Constant  Value=0
  OutRL Extend : Constant  Value=0
  OutRL Retract1 : Constant  Value=0
  OutRR Extend : Constant  Value=0
  OutRR Retract : Constant  Value=0
  Subtract BasketR : Sum  Inputs=+-
  Subtract Extend : Sum  Inputs=+-
  Subtract Jib : Sum  Inputs=+-
  Subtract Lift : Sum  Inputs=+-
  Subtract OutAll : Sum  Inputs=+-
  Subtract OutFL : Sum  Inputs=+-
  Subtract OutFR : Sum  Inputs=+-
  Subtract OutRL : Sum  Inputs=+-
  Subtract OutRR : Sum  Inputs=+-
  Subtract Tilt : Sum  Inputs=+-
  Subtract Track : Sum  Inputs=+-
  Subtract Turret : Sum  Inputs=+-
  Sum{1..4} (4 alike) : Sum  Inputs=++|
  Telescope Extend : Constant  Value=0
  Telescope Retract : Constant  Value=0
  Terminator1 : Terminator
  Tilt Down : Constant  Value=0
  Tilt Up : Constant  Value=0
  Track Extend : Constant  Value=0
  Track Retract : Constant  Value=0
  Turret Left : Constant  Value=0
  Turret Right : Constant  Value=0
  Out Bus Element : Outport  PortName=L  Element=Turret
  Out Bus Element1 : Outport  PortName=L  Element=Lift
  Out Bus Element2 : Outport  PortName=L  Element=Tilt
  Out Bus Element3 : Outport  PortName=L  Element=Jib
  Out Bus Element4 : Outport  PortName=L  Element=Extend
  Out Bus Element5 : Outport  PortName=L  Element=BasketR
  Out Bus Element6 : Outport  PortName=L  Element=OutRL
  Out Bus Element7 : Outport  PortName=L  Element=OutFL
  Out Bus Element8 : Outport  PortName=L  Element=TrackL
  Out Bus Element9 : Outport  PortName=L  Element=TrackR
  Out Bus Element10 : Outport  PortName=L  Element=OutRR
  Out Bus Element11 : Outport  PortName=L  Element=OutFR
  L1 : Outport  Port=2
  wires:
  Subtract OutAll/1 -> Sum1/1, Sum2/1, Sum3/1, Sum4/1
  OutAll Extend/1 -> Subtract OutAll/1  "Extend"
  OutAll Retract/1 -> Subtract OutAll/2  "Retract"
  Subtract OutRR/1 -> Sum4/2
  OutRR Extend/1 -> Subtract OutRR/1  "Extend"
  OutRR Retract/1 -> Subtract OutRR/2  "Retract"
  Subtract OutRL/1 -> Sum3/2
  OutRL Retract1/1 -> Subtract OutRL/2  "Retract"
  OutRL Extend/1 -> Subtract OutRL/1  "Extend"
  Subtract OutFL/1 -> Sum1/2
  Subtract OutFR/1 -> Sum2/2
  OutFR Extend/1 -> Subtract OutFR/1  "Extend"
  OutFR Retract/1 -> Subtract OutFR/2  "Retract"
  OutFL Retract1/1 -> Subtract OutFL/2  "Retract"
  OutFL Extend/1 -> Subtract OutFL/1  "Extend"
  Jib Extend/1 -> Subtract Jib/1  "Extend"
  Jib Retract/1 -> Subtract Jib/2  "Retract"
  Basket Right/1 -> Subtract BasketR/2  "Right"
  Basket Left/1 -> Subtract BasketR/1  "Left"
  Telescope Extend/1 -> Subtract Extend/1  "Extend"
  Telescope Retract/1 -> Subtract Extend/2  "Retract"
  Tilt Down/1 -> Subtract Tilt/2  "Down"
  Tilt Up/1 -> Subtract Tilt/1  "Up"
  Turret Left/1 -> Subtract Turret/1  "Left"
  Turret Right/1 -> Subtract Turret/2  "Right"
  Mux/1 -> Out Bus Element9/1  "TrackR"
  Track Extend/1 -> Subtract Track/1  "Extend"
  Track Retract/1 -> Subtract Track/2  "Retract"
  Bus Selector/1 -> Terminator1/1, L1/1  "<Jib Align>"
  S/1 -> Bus Selector/1
  Lift Down/1 -> Subtract Lift/2  "Down"
  Lift Up/1 -> Subtract Lift/1  "Up"
  Subtract Extend/1 -> Out Bus Element4/1  "Extend"
  Subtract Turret/1 -> Out Bus Element/1  "Turret"
  Subtract Lift/1 -> Out Bus Element1/1  "Lift"
  Subtract Tilt/1 -> Out Bus Element2/1  "Tilt"
  Sum1/1 -> Out Bus Element7/1  "OutFL"
  Subtract BasketR/1 -> Out Bus Element5/1  "BasketR"
  Subtract Jib/1 -> Out Bus Element3/1  "Jib"
  Sum3/1 -> Out Bus Element6/1  "OutRL"
  Sum2/1 -> Out Bus Element11/1  "OutFR"
  Sum4/1 -> Out Bus Element10/1  "OutRR"
  Subtract Track/1 -> Out Bus Element8/1, Mux/1  "TrackL"

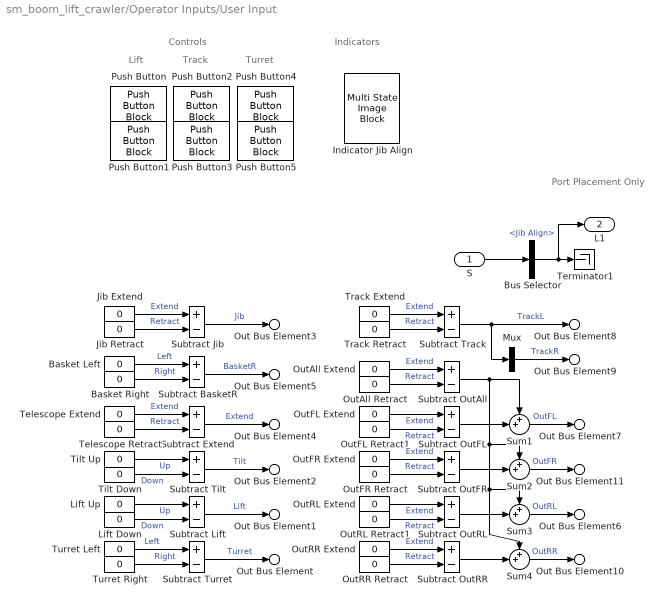
== system sm_boom_lift_crawler/Operator Inputs/User Input ==
  note: Controls
  note: Lift
  note: Port
      | Placement
      | Only
  note: Track
  note: Turret
  note: Indicators
  S : Inport
  Basket Left : Constant  Value=0
  Basket Right : Constant  Value=0
  Bus Selector : BusSelector  OutputSignals=Jib Align
  Indicator Jib Align : MultiStateImageBlock
  Jib Extend : Constant  Value=0
  Jib Retract : Constant  Value=0
  Lift Down : Constant  Value=0
  Lift Up : Constant  Value=0
  Mux : Mux  Inputs=1
  OutAll Extend : Constant  Value=0
  OutAll Retract : Constant  Value=0
  OutFL Extend : Constant  Value=0
  OutFL Retract1 : Constant  Value=0
  OutFR Extend : Constant  Value=0
  OutFR Retract : Constant  Value=0
  OutRL Extend : Constant  Value=0
  OutRL Retract1 : Constant  Value=0
  OutRR Extend : Constant  Value=0
  OutRR Retract : Constant  Value=0
  Push Button : PushButtonBlock  ButtonText=Up  IconOnColor=[0.0, 0.39215686274509803, 0.0]  IconOffColor=[0.0, 1.0, 0.0]
  Push Button1 : PushButtonBlock  ButtonText=Down  IconOnColor=[0.0, 0.39215686274509803, 0.0]  IconOffColor=[0.0, 1.0, 0.0]
  Push Button2 : PushButtonBlock  ButtonText=Out  IconOnColor=[0.0, 0.39215686274509803, 0.0]  IconOffColor=[0.0, 1.0, 0.0]
  Push Button3 : PushButtonBlock  ButtonText=In  IconOnColor=[0.0, 0.39215686274509803, 0.0]  IconOffColor=[0.0, 1.0, 0.0]
  Push Button4 : PushButtonBlock  ButtonText=L  IconOnColor=[0.0, 0.39215686274509803, 0.0]  IconOffColor=[0.0, 1.0, 0.0]
  Push Button5 : PushButtonBlock  ButtonText=R  IconOnColor=[0.0, 0.39215686274509803, 0.0]  IconOffColor=[0.0, 1.0, 0.0]
  Subtract BasketR : Sum  Inputs=+-
  Subtract Extend : Sum  Inputs=+-
  Subtract Jib : Sum  Inputs=+-
  Subtract Lift : Sum  Inputs=+-
  Subtract OutAll : Sum  Inputs=+-
  Subtract OutFL : Sum  Inputs=+-
  Subtract OutFR : Sum  Inputs=+-
  Subtract OutRL : Sum  Inputs=+-
  Subtract OutRR : Sum  Inputs=+-
  Subtract Tilt : Sum  Inputs=+-
  Subtract Track : Sum  Inputs=+-
  Subtract Turret : Sum  Inputs=+-
  Sum{1..4} (4 alike) : Sum  Inputs=++|
  Telescope Extend : Constant  Value=0
  Telescope Retract : Constant  Value=0
  Terminator1 : Terminator
  Tilt Down : Constant  Value=0
  Tilt Up : Constant  Value=0
  Track Extend : Constant  Value=0
  Track Retract : Constant  Value=0
  Turret Left : Constant  Value=0
  Turret Right : Constant  Value=0
  Out Bus Element : Outport  PortName=L  Element=Turret
  Out Bus Element1 : Outport  PortName=L  Element=Lift
  Out Bus Element2 : Outport  PortName=L  Element=Tilt
  Out Bus Element3 : Outport  PortName=L  Element=Jib
  Out Bus Element4 : Outport  PortName=L  Element=Extend
  Out Bus Element5 : Outport  PortName=L  Element=BasketR
  Out Bus Element6 : Outport  PortName=L  Element=OutRL
  Out Bus Element7 : Outport  PortName=L  Element=OutFL
  Out Bus Element8 : Outport  PortName=L  Element=TrackL
  Out Bus Element9 : Outport  PortName=L  Element=TrackR
  Out Bus Element10 : Outport  PortName=L  Element=OutRR
  Out Bus Element11 : Outport  PortName=L  Element=OutFR
  L1 : Outport  Port=2
  wires:
  Subtract Track/1 -> Mux/1, Out Bus Element8/1  "TrackL"
  Sum4/1 -> Out Bus Element10/1  "OutRR"
  Sum2/1 -> Out Bus Element11/1  "OutFR"
  Sum3/1 -> Out Bus Element6/1  "OutRL"
  Subtract Jib/1 -> Out Bus Element3/1  "Jib"
  Subtract BasketR/1 -> Out Bus Element5/1  "BasketR"
  Sum1/1 -> Out Bus Element7/1  "OutFL"
  Subtract Tilt/1 -> Out Bus Element2/1  "Tilt"
  Subtract Lift/1 -> Out Bus Element1/1  "Lift"
  Subtract Turret/1 -> Out Bus Element/1  "Turret"
  Subtract Extend/1 -> Out Bus Element4/1  "Extend"
  Lift Up/1 -> Subtract Lift/1  "Up"
  Lift Down/1 -> Subtract Lift/2  "Down"
  S/1 -> Bus Selector/1
  Bus Selector/1 -> L1/1, Terminator1/1  "<Jib Align>"
  Track Retract/1 -> Subtract Track/2  "Retract"
  Track Extend/1 -> Subtract Track/1  "Extend"
  Mux/1 -> Out Bus Element9/1  "TrackR"
  Turret Right/1 -> Subtract Turret/2  "Right"
  Turret Left/1 -> Subtract Turret/1  "Left"
  Tilt Up/1 -> Subtract Tilt/1  "Up"
  Tilt Down/1 -> Subtract Tilt/2  "Down"
  Telescope Retract/1 -> Subtract Extend/2  "Retract"
  Telescope Extend/1 -> Subtract Extend/1  "Extend"
  Basket Left/1 -> Subtract BasketR/1  "Left"
  Basket Right/1 -> Subtract BasketR/2  "Right"
  Jib Retract/1 -> Subtract Jib/2  "Retract"
  Jib Extend/1 -> Subtract Jib/1  "Extend"
  OutFL Extend/1 -> Subtract OutFL/1  "Extend"
  OutFL Retract1/1 -> Subtract OutFL/2  "Retract"
  OutFR Retract/1 -> Subtract OutFR/2  "Retract"
  OutFR Extend/1 -> Subtract OutFR/1  "Extend"
  Subtract OutFR/1 -> Sum2/2
  Subtract OutFL/1 -> Sum1/2
  OutRL Extend/1 -> Subtract OutRL/1  "Extend"
  OutRL Retract1/1 -> Subtract OutRL/2  "Retract"
  Subtract OutRL/1 -> Sum3/2
  OutRR Retract/1 -> Subtract OutRR/2  "Retract"
  OutRR Extend/1 -> Subtract OutRR/1  "Extend"
  Subtract OutRR/1 -> Sum4/2
  OutAll Retract/1 -> Subtract OutAll/2  "Retract"
  OutAll Extend/1 -> Subtract OutAll/1  "Extend"
  Subtract OutAll/1 -> Sum4/1, Sum3/1, Sum2/1, Sum1/1

== system sm_boom_lift_crawler/Control/Hold/Deviator Valve Commands ==
  Constant : Constant
  Constant1 : Constant  Value=-1
  Bus Element Out14 : Outport  VectorParamsAs1DForOutWhenUnconnected=off  PortName=Dev  Element=g
  Bus Element Out15 : Outport  VectorParamsAs1DForOutWhenUnconnected=off  PortName=Dev  Element=s
  wires:
  Constant/1 -> Bus Element Out14/1
  Constant1/1 -> Bus Element Out15/1

== system sm_boom_lift_crawler/Control/Hold/Ground Valve Commands ==
  Constant : Constant
  Constant1 : Constant  Value=0
  Constant2 : Constant  Value=0
  Bus Element Out1 : Outport  VectorParamsAs1DForOutWhenUnconnected=off  PortName=Gnd  Element=Pr
  Bus Element Out : Outport  VectorParamsAs1DForOutWhenUnconnected=off  PortName=Gnd  Element=Ou
  Bus Element Out2 : Outport  VectorParamsAs1DForOutWhenUnconnected=off  PortName=Gnd  Element=Tr
  wires:
  Constant/1 -> Bus Element Out1/1
  Constant1/1 -> Bus Element Out/1
  Constant2/1 -> Bus Element Out2/1

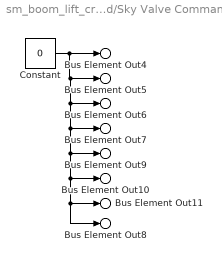
== system sm_boom_lift_crawler/Control/Hold/Sky Valve Commands ==
  Constant : Constant  Value=0
  Bus Element Out4 : Outport  VectorParamsAs1DForOutWhenUnconnected=off  PortName=Sky  Element=Pr
  Bus Element Out5 : Outport  VectorParamsAs1DForOutWhenUnconnected=off  PortName=Sky  Element=Tu
  Bus Element Out6 : Outport  VectorParamsAs1DForOutWhenUnconnected=off  PortName=Sky  Element=Li
  Bus Element Out7 : Outport  VectorParamsAs1DForOutWhenUnconnected=off  PortName=Sky  Element=Ti
  Bus Element Out8 : Outport  VectorParamsAs1DForOutWhenUnconnected=off  PortName=Sky  Element=BL
  Bus Element Out9 : Outport  VectorParamsAs1DForOutWhenUnconnected=off  PortName=Sky  Element=Ex
  Bus Element Out10 : Outport  VectorParamsAs1DForOutWhenUnconnected=off  PortName=Sky  Element=Ji
  Bus Element Out11 : Outport  VectorParamsAs1DForOutWhenUnconnected=off  PortName=Sky  Element=BR
  wires:
  Constant/1 -> Bus Element Out4/1, Bus Element Out7/1, Bus Element Out9/1, Bus Element Out10/1, Bus Element Out11/1, Bus Element Out8/1, Bus Element Out6/1, Bus Element Out5/1

== system sm_boom_lift_crawler/Control/Valve Sequence/Deviator Valve Commands ==
  In Bus Element3 : Inport  PortName=t
  In Bus Element4 : Inport  PortName=t
  Ground Deviator Valve : Subsystem
  Sky Deviator Valve : Subsystem
  Bus Element Out14 : Outport  VectorParamsAs1DForOutWhenUnconnected=off  PortName=Dev  Element=g
  Bus Element Out15 : Outport  VectorParamsAs1DForOutWhenUnconnected=off  PortName=Dev  Element=s
  wires:
  In Bus Element4/1 -> Ground Deviator Valve/1(t)
  Ground Deviator Valve/1(C) -> Bus Element Out14/1
  In Bus Element3/1 -> Sky Deviator Valve/1(t)
  Sky Deviator Valve/1(C) -> Bus Element Out15/1

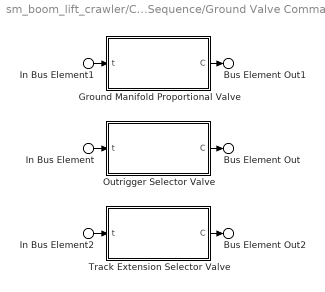
== system sm_boom_lift_crawler/Control/Valve Sequence/Ground Valve Commands ==
  In Bus Element : Inport  PortName=t
  In Bus Element1 : Inport  PortName=t
  In Bus Element2 : Inport  PortName=t
  Ground Manifold Proportional Valve : Subsystem
  Outrigger Selector Valve : Subsystem
  Track Extension Selector Valve : Subsystem
  Bus Element Out1 : Outport  VectorParamsAs1DForOutWhenUnconnected=off  PortName=Gnd  Element=Pr
  Bus Element Out : Outport  VectorParamsAs1DForOutWhenUnconnected=off  PortName=Gnd  Element=Ou
  Bus Element Out2 : Outport  VectorParamsAs1DForOutWhenUnconnected=off  PortName=Gnd  Element=Tr
  wires:
  In Bus Element/1 -> Outrigger Selector Valve/1(t)
  Track Extension Selector Valve/1(C) -> Bus Element Out2/1
  Ground Manifold Proportional Valve/1(C) -> Bus Element Out1/1
  In Bus Element2/1 -> Track Extension Selector Valve/1(t)
  In Bus Element1/1 -> Ground Manifold Proportional Valve/1(t)
  Outrigger Selector Valve/1(C) -> Bus Element Out/1

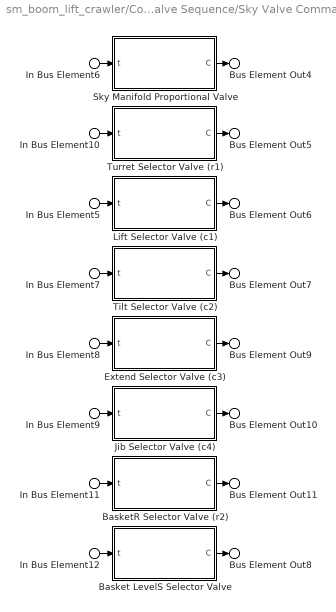
== system sm_boom_lift_crawler/Control/Valve Sequence/Sky Valve Commands ==
  In Bus Element{5..12} (8 alike) : Inport  PortName=t
  Basket LevelS Selector Valve : Subsystem
  BasketR Selector Valve (r2) : Subsystem
  Extend Selector Valve (c3) : Subsystem
  Jib Selector Valve (c4) : Subsystem
  Lift Selector Valve (c1) : Subsystem
  Sky Manifold Proportional Valve : Subsystem
  Tilt Selector Valve (c2) : Subsystem
  Turret Selector Valve (r1) : Subsystem
  Bus Element Out4 : Outport  VectorParamsAs1DForOutWhenUnconnected=off  PortName=Sky  Element=Pr
  Bus Element Out5 : Outport  VectorParamsAs1DForOutWhenUnconnected=off  PortName=Sky  Element=Tu
  Bus Element Out6 : Outport  VectorParamsAs1DForOutWhenUnconnected=off  PortName=Sky  Element=Li
  Bus Element Out7 : Outport  VectorParamsAs1DForOutWhenUnconnected=off  PortName=Sky  Element=Ti
  Bus Element Out8 : Outport  VectorParamsAs1DForOutWhenUnconnected=off  PortName=Sky  Element=BL
  Bus Element Out9 : Outport  VectorParamsAs1DForOutWhenUnconnected=off  PortName=Sky  Element=Ex
  Bus Element Out10 : Outport  VectorParamsAs1DForOutWhenUnconnected=off  PortName=Sky  Element=Ji
  Bus Element Out11 : Outport  VectorParamsAs1DForOutWhenUnconnected=off  PortName=Sky  Element=BR
  wires:
  In Bus Element10/1 -> Turret Selector Valve (r1)/1(t)
  BasketR Selector Valve (r2)/1(C) -> Bus Element Out11/1
  Extend Selector Valve (c3)/1(C) -> Bus Element Out9/1
  Jib Selector Valve (c4)/1(C) -> Bus Element Out10/1
  In Bus Element11/1 -> BasketR Selector Valve (r2)/1(t)
  Turret Selector Valve (r1)/1(C) -> Bus Element Out5/1
  In Bus Element12/1 -> Basket LevelS Selector Valve/1(t)
  Sky Manifold Proportional Valve/1(C) -> Bus Element Out4/1
  Basket LevelS Selector Valve/1(C) -> Bus Element Out8/1
  Lift Selector Valve (c1)/1(C) -> Bus Element Out6/1
  In Bus Element6/1 -> Sky Manifold Proportional Valve/1(t)
  In Bus Element5/1 -> Lift Selector Valve (c1)/1(t)
  In Bus Element7/1 -> Tilt Selector Valve (c2)/1(t)
  Tilt Selector Valve (c2)/1(C) -> Bus Element Out7/1
  In Bus Element9/1 -> Jib Selector Valve (c4)/1(t)
  In Bus Element8/1 -> Extend Selector Valve (c3)/1(t)

== system sm_boom_lift_crawler/Control/Valve Sequence/Deviator Valve Commands/Ground Deviator Valve ==
  t : Inport
  Selector Valve Input : Lookup_n-D  NumberOfTableDimensions=1  BreakpointsForDimension1=tVec.deviators.ground  Table=oVec.deviators.ground  InterpMethod=Flat  ExtrapMethod=Clip  UseLastTableValue=on  InternalRulePriority=Speed  RndMeth=Simplest
  C : Outport
  wires:
  Selector Valve Input/1 -> C/1
  t/1 -> Selector Valve Input/1

== system sm_boom_lift_crawler/Control/Valve Sequence/Deviator Valve Commands/Sky Deviator Valve ==
  t : Inport
  Selector Valve Input : Lookup_n-D  NumberOfTableDimensions=1  BreakpointsForDimension1=tVec.deviators.sky  Table=oVec.deviators.sky  InterpMethod=Flat  ExtrapMethod=Clip  UseLastTableValue=on  InternalRulePriority=Speed  RndMeth=Simplest
  C : Outport
  wires:
  t/1 -> Selector Valve Input/1
  Selector Valve Input/1 -> C/1

== system sm_boom_lift_crawler/Control/Valve Sequence/Ground Valve Commands/Ground Manifold Proportional Valve ==
  t : Inport
  Selector Valve Input : Lookup_n-D  NumberOfTableDimensions=1  BreakpointsForDimension1=tVec.ground.proportional  Table=oVec.ground.proportional  InterpMethod=Flat  ExtrapMethod=Clip  UseLastTableValue=on  InternalRulePriority=Speed  RndMeth=Simplest
  C : Outport
  wires:
  Selector Valve Input/1 -> C/1
  t/1 -> Selector Valve Input/1

== system sm_boom_lift_crawler/Control/Valve Sequence/Ground Valve Commands/Outrigger Selector Valve ==
  t : Inport
  Selector Valve Input : Lookup_n-D  NumberOfTableDimensions=1  BreakpointsForDimension1=tVec.ground.c1.all  Table=oVec.ground.c1.all  InterpMethod=Flat  ExtrapMethod=Clip  UseLastTableValue=on  InternalRulePriority=Speed  RndMeth=Simplest
  C : Outport
  wires:
  t/1 -> Selector Valve Input/1
  Selector Valve Input/1 -> C/1

== system sm_boom_lift_crawler/Control/Valve Sequence/Ground Valve Commands/Track Extension Selector Valve ==
  t : Inport
  Selector Valve Input : Lookup_n-D  NumberOfTableDimensions=1  BreakpointsForDimension1=tVec.ground.c5.all  Table=oVec.ground.c5.all  InterpMethod=Flat  ExtrapMethod=Clip  UseLastTableValue=on  InternalRulePriority=Speed  RndMeth=Simplest
  C : Outport
  wires:
  Selector Valve Input/1 -> C/1
  t/1 -> Selector Valve Input/1
